simulink model "Copy_3_of_trial_with_intermediate_tanks"  (R2024b)
settings: Solver=ode15s  StartTime=0.0  StopTime=0.1  FixedStep=1e-7  MaxStep=1e-6  RelTol=1e-6
InitFcn:
  | param = struct();
  | 
  | % Fluid Properties
  | param.rho = 870;
  | 
  | % Pressure Rails
  | param.P_H = 20e6;
  | param.P_M = 10e6;
  | param.P_L = 101325;
  | 
  | % Linear Actuator Chamber
  | param.V1_0 = 100e-6;
  | param.Acap = pi*(0.5*2.54)^2*1e-4;
  | 
  | % Intermediary volumes
  | param.V3_0 = 25e-6;
  | param.V4_0 = 25e-6;
  | 
  | % Fluid
  | param.beta = 1.8e9;
  | param.air = 0.05;
  | 
  | % Valve
  | param.max_Avt = 0.5*0.25*pi*(20e-3)^2;
  | param.Cd = 0.6;
  | 
  | % Valve Dynamics
  | param.wn = 50*2*pi;
  | param.zeta = 1;
  | 
  | % Hydraulic Pump/Motor
  | param.J_hyd = 3000e-7;
  | param.D = 0.8e-6;    % In cc/rev
  | 
  | % Electric Motor/Generator
  | param.J_elec = 3060e-7;
  | param.Kt = 109e-3;
settings Model: Creator=ibrah408  LastModifiedBy=user
settings SolverCC: MaxConsecutiveZCs=10000
settings RTWCC: GPUComputeCapability=3.5

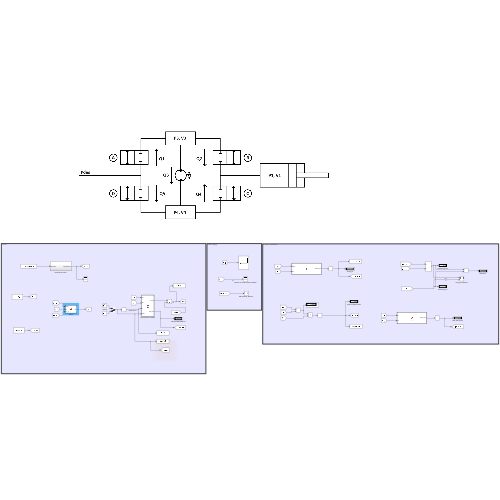
[thumbnail: Simulink's stored preview of the top-level diagram]
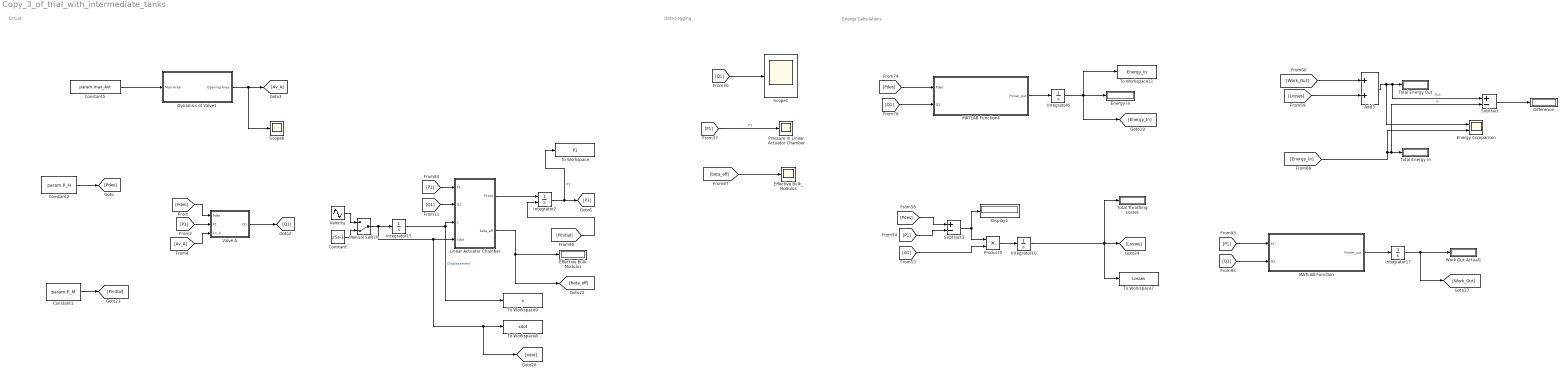
== system Copy_3_of_trial_with_intermediate_tanks ==
  note: Energy Calculations
  note: Data Logging
  note: Circuit
  Add3 : Sum
  Constant : Constant  Value=25e-3
  Constant1 : Constant  Value=param.P_M
  Constant2 : Constant  Value=param.P_H
  Constant5 : Constant  Value=param.max_Avt
  Difference : Display
  Display4 : Display
  Dynamics of Valve1 : Subsystem
  Effective Bulk Modulus : Display
  Effective Bulk_Modulus : Scope
  Energy Comparison : Scope  NumInputPorts=2
  Energy In : Display
  Integrator{6,10,15,17} (4 alike) : Integrator
  Integrator2 : Integrator  InitialConditionSource=external  InitialCondition=param.P_M
  Linear Actuator Chamber : MATLAB Function  TreatAsAtomicUnit=on
  MATLAB Function : MATLAB Function  TreatAsAtomicUnit=on
  MATLAB Function4 : MATLAB Function  TreatAsAtomicUnit=on
  Manual Switch : ManualSwitch  CurrentSetting=0
  Pressure in Linear Actuator Chamber : Scope
  Product5 : Product
  Scope1 : Scope
  Scope6 : Scope
  Subtract : Sum  Inputs=+-
  Subtract3 : Sum  Inputs=+-
  To Workspace : ToWorkspace  VariableName=P1  SaveFormat=Timeseries  SampleTime=-1
  To Workspace11 : ToWorkspace  VariableName=Energy_In  SaveFormat=Timeseries  SampleTime=-1
  To Workspace7 : ToWorkspace  VariableName=Losses  SaveFormat=Timeseries  SampleTime=-1
  To Workspace8 : ToWorkspace  VariableName=xdot  SaveFormat=Timeseries  SampleTime=-1
  To Workspace9 : ToWorkspace  VariableName=x  SaveFormat=Timeseries  SampleTime=-1
  Total Energy In : Display
  Total Energy Out : Display
  Total Throttling Losses : Display
  Valve A : MATLAB Function  TreatAsAtomicUnit=on
  Velocity : Sin  Amplitude=1e-2  Frequency=(2*pi)/0.2  Phase=pi/2  SampleTime=0
  Work Out Actual1 : Display
  wires:
  [Pdes] -> Valve A/1(Pdes)
  Constant2/1 -> [Pdes]
  [P1] -> Valve A/2(P1)
  Valve A/1(Q1) -> [Q1]
  [Av_A] -> Valve A/3(Av_A)
  Linear Actuator Chamber/1(P1dot) -> Integrator2/1
  [Pinitial] -> Integrator2/2
  Integrator2/1 -> To Workspace/1, [P1]  "P3"
  [Q1] -> Linear Actuator Chamber/2(Q1)
  [Q1] -> Scope1/1
  [P1] -> Pressure in Linear Actuator Chamber/1  "P1"
  Integrator6/1 -> To Workspace11/1, [Energy_In], Energy In/1
  Dynamics of Valve1/1(Opening Area) -> Scope6/1, [Av_A]
  Constant5/1 -> Dynamics of Valve1/1(Max Area)
  Subtract3/1 -> Display4/1, Product5/1
  [Pdes] -> Subtract3/1
  Integrator10/1 -> Total Throttling Losses/1, To Workspace7/1, [Losses]
  Product5/1 -> Integrator10/1
  [P1] -> Subtract3/2
  [Q1] -> Product5/2
  [Work_Out] -> Add3/1
  [Losses] -> Add3/2
  [Energy_In] -> Energy Comparison/2, Subtract/2, Total Energy In/1  "In"
  Add3/1 -> Energy Comparison/1, Subtract/1, Total Energy Out/1  "Out"
  Integrator15/1 -> To Workspace9/1, Linear Actuator Chamber/3(x)  "Displacement"
  Velocity/1 -> Manual Switch/1
  Manual Switch/1 -> Integrator15/1, [xdot], To Workspace8/1, Linear Actuator Chamber/4(xdot)
  Constant/1 -> Manual Switch/2
  Linear Actuator Chamber/2(beta_eff) -> [beta_eff], Effective Bulk Modulus/1
  [P1] -> Linear Actuator Chamber/1(P1)
  [beta_eff] -> Effective Bulk_Modulus/1
  Constant1/1 -> [Pinitial]
  [Q1] -> MATLAB Function/2(Q1)
  [P1] -> MATLAB Function/1(P1)
  MATLAB Function/1(Power_out) -> Integrator17/1
  Integrator17/1 -> Work Out Actual1/1, [Work_Out]
  Subtract/1 -> Difference/1
  [Pdes] -> MATLAB Function4/1(Pdes)
  [Q1] -> MATLAB Function4/2(Q1)
  MATLAB Function4/1(Power_out) -> Integrator6/1

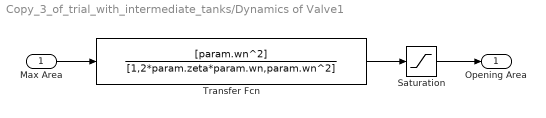
== system Copy_3_of_trial_with_intermediate_tanks/Dynamics of Valve1 ==
  Max Area : Inport
  Saturation : Saturate  UpperLimit=param.max_Avt  LowerLimit=0
  Transfer Fcn : TransferFcn  Numerator=[param.wn^2]  Denominator=[1,2*param.zeta*param.wn,param.wn^2]
  Opening Area : Outport
  wires:
  Max Area/1 -> Transfer Fcn/1
  Saturation/1 -> Opening Area/1
  Transfer Fcn/1 -> Saturation/1

== matlab function Copy_3_of_trial_with_intermediate_tanks/Valve A ==
  data: Pdes input; Q1 output; P1 input; Av_A input; param parameter
function Q1 = fcn(Pdes, P1, Av_A, param)

delP = Pdes - P1;
Q1 = (1/sqrt(2))*param.Cd*Av_A*sqrt(2/param.rho)*sqrt(abs(delP))*sign(delP);

== matlab function Copy_3_of_trial_with_intermediate_tanks/Linear Actuator Chamber ==
  data: P1 input; Q1 input; P1dot output; x input; xdot input; param parameter; beta_eff output
function [P1dot, beta_eff] = fcn(P1,Q1,x, xdot, param)

gamma = 1.4; % Adiabatic process
Pt = param.P_L;

Pg = P1-Pt;   % Gauge pressure
r = P1/Pt;    % Pressure ratio
e = exp(Pg/param.beta);
rv = (1/e+param.air*r^(-1/gamma))/(1+param.air);      %Volume ratio

% Note: beta_mix as calculated by Hans Barkei
beta_eff = rv*(1+param.air)/(1/(e*param.beta)+param.air/(gamma*Pt*r^(1/gamma+1)));

P1dot = (beta_eff/(param.V1_0+param.Acap*x))*(Q1-param.Acap*xdot);

== matlab function Copy_3_of_trial_with_intermediate_tanks/MATLAB Function4 ==
  data: Pdes input; Q1 input; Power_out output; param parameter
function Power_out = fcn(Pdes, Q1, param)

gamma = 1.4; % Adiabatic process
Pt = param.P_L;

Pg = Pdes-Pt;   % Gauge pressure
r = Pdes/Pt;    % Pressure ratio
e = exp(Pg/param.beta);
rv = (1/e+param.air*r^(-1/gamma))/(1+param.air);      %Volume ratio

El=param.beta*(e-(1+Pg/param.beta))+Pt*(e-1);           %Energy in liquid
Eg=Pdes/(gamma-1).*(1-r.^(1/gamma-1));          %Energy in gas
E=(El./e+param.air*Eg.*r.^(-1/gamma))./(1./e+param.air*r.^(-1/gamma));    %Energy in mixture
W = E-(1./rv-1)*Pt;  %Compressibility (volumetric) energy density

Power_out = (Q1)*(W+Pg);

== matlab function Copy_3_of_trial_with_intermediate_tanks/MATLAB Function ==
  data: P1 input; Q1 input; Power_out output; param parameter
function Power_out = fcn(P1, Q1, param)

gamma = 1.4; % Adiabatic process
Pt = param.P_L;

Pg = P1-Pt;   % Gauge pressure
r = P1/Pt;    % Pressure ratio
e = exp(Pg/param.beta);
rv = (1/e+param.air*r^(-1/gamma))/(1+param.air);      %Volume ratio

El=param.beta*(e-(1+Pg/param.beta))+Pt*(e-1);           %Energy in liquid
Eg=P1/(gamma-1).*(1-r.^(1/gamma-1));          %Energy in gas
E=(El./e+param.air*Eg.*r.^(-1/gamma))./(1./e+param.air*r.^(-1/gamma));    %Energy in mixture
W = E-(1./rv-1)*Pt;  %Compressibility (volumetric) energy density

Power_out = (Q1)*(W+Pg);
